simulink model "RT_AI"  (R2024b)
settings: Solver=ode1  StartTime=0.0  StopTime=3  FixedStep=Ts  RelTol=1e-3
PreLoadFcn:
  | Net_improve_init;L=Lac_MV;Tctrl=Ts;
PostLoadFcn:
  | Net_improve_init;L=Lac_MV;Tctrl=Ts;
InitFcn:
  | Net_improve_init;L=Lac_MV;Tctrl=Ts;
undefined symbols (not defined in the file): C1, dend, DiscIntNeverNeededParam, f_cari, fs, Lac_MV, numd, Pref, Rac_MV, Ts, Vac_peak_MV, Vdc
libraries: rtlab x6, spsControlledVoltageSourceLib x6, powerlib_extras x5, artemis x3, spsControlledCurrentSourceLib x3, spsGroundLib x3, simulink x3, spsCurrentMeasurementLib x2, spsThreePhaseVIMeasurementLib x1, spsIdealSwitchLib x1, spsPower3phInstantaneousLib x1, spsSeriesRLCBranchLib x1
Description:
  | The Model initialization function Callback automatically
  | 
  | sets the sample time  to 2e-6 sec.  and loads the initial
  | 
  | states vector xInitial. The initial state vector is saved in the
  | 
  | power_acdrive_init.mat file.
  | 
  | 
  | 
  | Check  the Initial state checkbox in the Simulation
  | 
  | parameters/Workspace I/O to start in steady state with a
  | 
  | speed of 120 rad/s and a torque of 0 N.m/s,
  | 
  | 
  | Copyright 2008-2015 The MathWorks, Inc.
settings Model: Creator=WeiLi  LastModifiedBy=KeXing
settings SolverCC: AlgebraicLoopSolver=TrustRegion
settings DataIOCC: SaveFinalState=on  SaveFormat=Array  SignalLoggingSaveFormat=ModelDataLogs  SaveOutput=off  SaveTime=off  ReturnWorkspaceOutputs=off  SignalLoggingName=sigsOut
settings OptimizationCC: BlockReduction=off  ExpressionDepthLimit=2147483647  InitFltsAndDblsToZero=on  LifeSpan=inf
settings DebuggingCC: SaveWithParameterizedLinksMsg=none  UnderspecifiedInitializationDetection=Classic  MergeDetectMultiDrivingBlocksExec=none  CheckExecutionContextPreStartOutputMsg=on  SignalResolutionControl=TryResolveAllWithWarning  MultiTaskDSMMsg=warning  MultiTaskCondExecSysMsg=none  FcnCallInpInsideContextMsg=warning  UnconnectedInputMsg=warning  UnconnectedLineMsg=warning  StateNameClashWarn=warning  SFUnexpectedBacktrackingDiag=warning  SFNoUnconditionalDefaultTransitionDiag=warning  SFExecutionAtInitializationDiag=none  ArithmeticOperatorsInVariantConditions=warning
settings HardwareCC: ProdBitPerPointer=32  ProdBitPerSizeT=32  ProdBitPerPtrDiffT=32  ProdLargestAtomicFloat=None  ProdIntDivRoundTo=Undefined  ProdEndianess=Unspecified  ProdWordSize=32  ProdHWDeviceType=32-bit Generic  TargetUnknown=on
settings ModelReferenceCC: EnableRefExpFcnMdlSchedulingChecks=on  PropagateSignalLabelsOutOfModel=off
settings SFSimCC: SimUseLocalCustomCode=off  CustomCodeUndefinedFunction=UseInterfaceOnly
settings RTWCC: RTWUseLocalCustomCode=off  GPUComputeCapability=3.5
settings CodeAppCC: StateflowObjectComments=on
settings GRTTargetCC: TargetFcnLib=ansi_tfl_tmw.mat  TargetLangStandard=C89/C90 (ANSI)  CombineOutputUpdateFcns=off  GRTInterface=on
settings ConfigComp: CovMetricSettings=dw  CovSaveCumulativeToWorkspaceVar=on  CovSaveSingleToWorkspaceVar=on  CovExternalEMLEnable=off
settings SimscapeCC: SimscapeNormalizeSystem=off

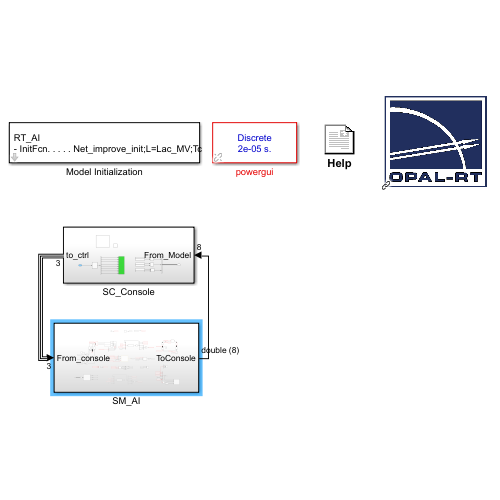
[thumbnail: Simulink's stored preview of the top-level diagram]
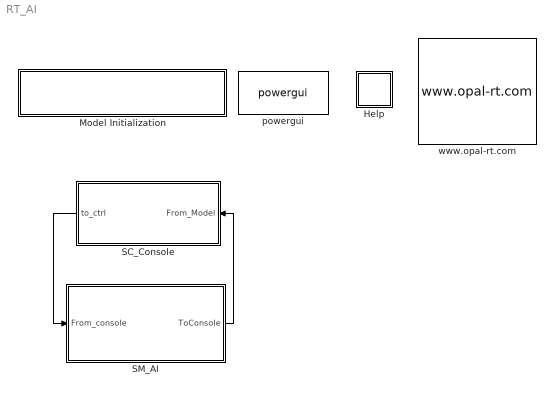
== system RT_AI ==
  Help : Subsystem  mask(OpDoc){docfile=../Help/help.html}
      mask init:
      | %patch([1,1,0,0,.8,1],[.8,0,0,1,1,.8],[.8 .8 .8]);
      | %patch([.15 .78 .78 .15 .15],[.8 .8 .83 .83 .8],[.9 .9 .9]);
      | %patch([.15 .78 .78 .15 .15],[.7 .7 .73 .73 .8],[.9 .9 .9]);
      | %patch([.15 .78 .78 .15 .15],[.6 .6 .63 .63 .6],[.9 .9 .9]);
      | %patch([.15 .78 .78 .15 .15],[.5 .5 .53 .53 .5],[.9 .9 .9]);
      | %patch([.15 .78 .78 .15 .15],[.4 .4 .43 .43 .4],[.9 .9 .9]);
      settings: OpenFcn=OpHelp_cb(gcb);
      mask Display: image(imread('opdoc.bmp'))
  Model Initialization : Subsystem  mask(Model Functions){InitFcnX=Net_improve_init;L=Lac_MV;Tctrl=Ts;, prel=on, posl=on, inif=on, strf=off}
      mask prompts: InitFcnX "Initialisation"; prel "Preload Function"; posl "PostLoad Function"; inif "InitFcn"; strf "StartFcn"
      mask init:
      | currentBlock = gcb;
      | root = bdroot(currentBlock);
      | 
      | if ~strcmp(get_param(root,'BlockDiagramType'),'library')
      |     if prel==1
      |         set_param(root, 'PreLoadFcn', InitFcnX);
      |     else
      |         set_param(root, 'PreLoadFcn', '');
      |     end
      |     if inif==1
      |         set_param(root, 'InitFcn', InitFcnX);
      |     else
      |         set_param(root, 'InitFcn', '');
      |     end
      |     if strf==1
      |         set_param(root, 'StartFcn', InitFcnX);
      |     else
      |         set_param(root, 'StartFcn', '');
      |     end
      |     if posl==1
      |         set_param(root, 'PostLoadFcn', InitFcnX);
      |     else
      |         set_param(root, 'PostLoadFcn', '');
      |     end
      | end
      | 
      | pos = get_param(currentBlock, 'Position');
      | width = pos(3) - pos(1); height = pos(4) - pos(2);
      | txt = [ upper(root) '\n' '- InitFcn. . . . . '  get_param(root, 'InitFcn') ];
      settings: CopyFcn=set_param(gcb,'LinkStatus','none')
      mask Display: text(5, height*0.5, txt, 'horizontalAlignment', 'left', 'verticalAlignment', 'middle') ;
  SC_Console : Subsystem
  SM_AI : Subsystem
  powergui : sps_lib/powergui  Priority=2  SimulationMode=Discrete  SampleTime=Ts  frequency=60  Iterations=50  frequencyindice=0  Pbase=100e6  ErrMax=1e-4  UnitsV=kV  UnitsW=MW  buscounter=0  FunctionMessages=off  echomessages=off  EnableUseOfTLC=off  CurrentSourceSwitches=off  DisableSnubberDevices=off  DisableRonSwitches=off  DisableVfSwitches=off  DisplayEquations=off  AutomaticDiscreteSolvers=off  SolverType=Backward Euler  Interpol=off  ExternalGateDelay=off  methode=off  Ts=0  x0status=blocks  SPID=off  SwTol=0  HookPort=off  NonlinearTolerance=1e-4  nMaxIteration=100  ContinueOnMaxIteration=off  RestoreLinks=warning  ResistiveCurrentMeasurement=off  Frange=[0:2:500]  Ylog=off  Xlog=on  ShowGrid=off  save=off  variable=ZData  structure=VI  ZoomFFT=off  StartTime=9  cycles=10  DisplayStyle=2  fundamental=300/pi  FreqAxis=off  MaxFrequency=1000  frequencyindicesteady=1  RmsSteady=1  display=off
  www.opal-rt.com : artemis/Internal/www.opal-rt.com  SystemSampleTime=-1  VariantActivationTime=update diagram  AllowFlexibleInterface=on  Latency=0  AutoFrameSizeCalculation=off
      settings: SourceProductName=Artemis
  wires:
  SC_Console/1(to_ctrl) -> SM_AI/1(From_console)
  SM_AI/1(ToConsole) -> SC_Console/1(From_Model)

== system RT_AI/Help ==

== system RT_AI/Model Initialization ==

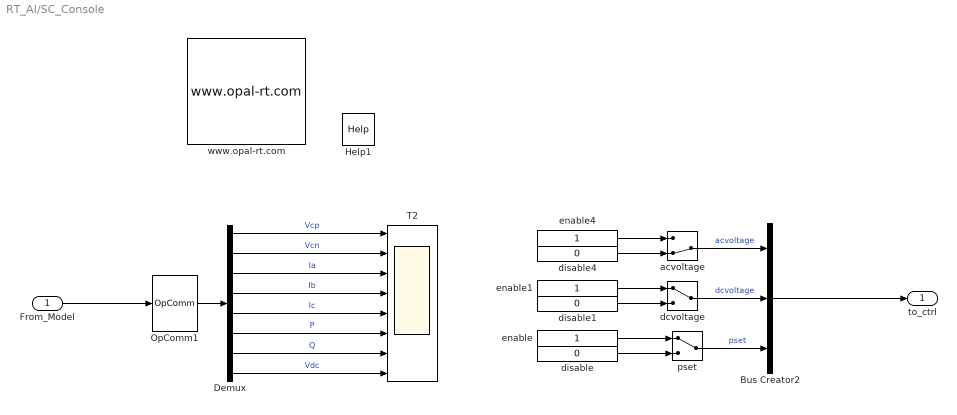
== system RT_AI/SC_Console ==
  From_Model : Inport
  Bus Creator2 : BusCreator  Inputs=3
  Demux : Demux  Outputs=8
  Help1 : artemis/Internal/Help  docfile=../help/help.html
      settings: SourceProductName=Artemis
  OpComm1 : rtlab/OpComm  nbport=1  groupe_acq=1  subsys_rate=Ts  st=0  Synchronization=off  Interpolation=on  Threshold=1.0  Missed_Data=off  Sim_Time=off  Samples=off  dynSigOut=off  from_console=0  warning_done=off  writeOpCommFile=off  Offset=off
      settings: SourceProductName=RT-LAB
  T2 : Scope  NumInputPorts=8
  acvoltage : ManualSwitch  CurrentSetting=0
  dcvoltage : ManualSwitch
  disable : Constant  Value=0
  disable1 : Constant  Value=0
  disable4 : Constant  Value=0
  enable : Constant
  enable1 : Constant
  enable4 : Constant
  pset : ManualSwitch
  www.opal-rt.com : artemis/Internal/www.opal-rt.com  SystemSampleTime=-1  VariantActivationTime=update diagram  AllowFlexibleInterface=on  Latency=0  AutoFrameSizeCalculation=off
      settings: SourceProductName=Artemis
  to_ctrl : Outport
  wires:
  enable/1 -> pset/1
  Bus Creator2/1 -> to_ctrl/1
  dcvoltage/1 -> Bus Creator2/2  "dcvoltage"
  disable1/1 -> dcvoltage/2
  disable/1 -> pset/2
  enable1/1 -> dcvoltage/1
  disable4/1 -> acvoltage/2
  enable4/1 -> acvoltage/1
  acvoltage/1 -> Bus Creator2/1  "acvoltage"
  pset/1 -> Bus Creator2/3  "pset"
  Demux/1 -> T2/1  "Vcp"
  Demux/6 -> T2/6  "P"
  From_Model/1 -> OpComm1/1
  Demux/2 -> T2/2  "Vcn"
  OpComm1/1 -> Demux/1
  Demux/3 -> T2/3  "Ia"
  Demux/8 -> T2/8  "Vdc"
  Demux/4 -> T2/4  "Ib"
  Demux/5 -> T2/5  "Ic"
  Demux/7 -> T2/7  "Q"

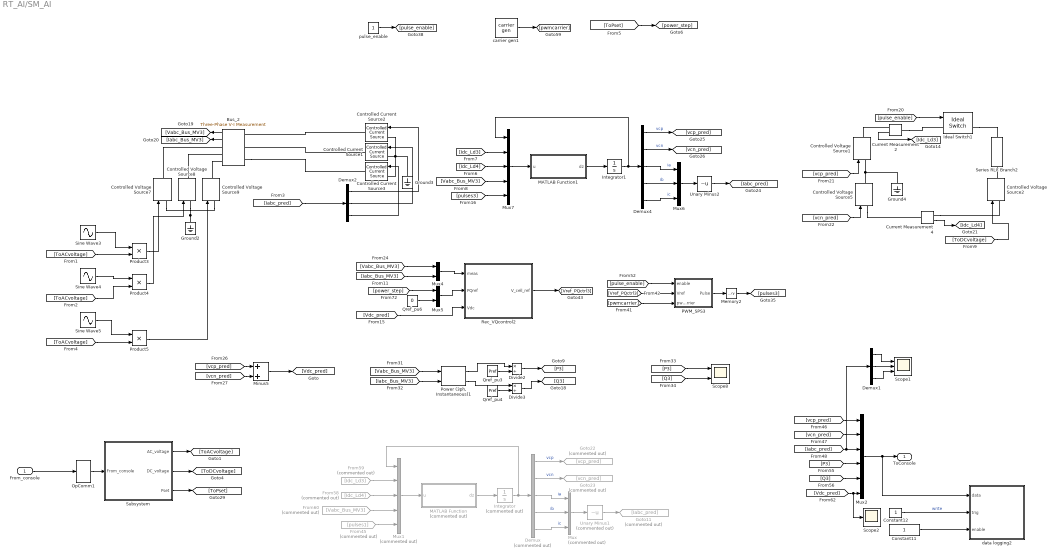
== system RT_AI/SM_AI ==
  From_console : Inport
  Bus_2 : spsThreePhaseVIMeasurementLib/Three-Phase V-I Measurement  VoltageMeasurement=phase-to-ground  SetLabelV=off  LabelV=Vabc  Vpu=off  VpuLL=off  CurrentMeasurement=yes  SetLabelI=off  LabelI=Iabc  Ipu=off  Pbase=P_AC  Vbase=V_AC_prim  OutputType=Complex  PhasorSimulation=off  PSBequivalent=0
  Constant11 : Constant
  Constant12 : Constant
  Controlled Current Source1 : spsControlledCurrentSourceLib/Controlled Current Source  Initialize=on  Source_Type=AC  Amplitude=0  Phase=0  Frequency=0  Measurements=None
  Controlled Current Source2 : spsControlledCurrentSourceLib/Controlled Current Source  Initialize=on  Source_Type=AC  Amplitude=0  Phase=0  Frequency=0  Measurements=None
  Controlled Current Source3 : spsControlledCurrentSourceLib/Controlled Current Source  Initialize=on  Source_Type=AC  Amplitude=0  Phase=0  Frequency=0  Measurements=None
  Controlled Voltage Source1 : spsControlledVoltageSourceLib/Controlled Voltage Source  Initialize=on  Source_Type=DC  Amplitude=3000  Phase=0  Frequency=0  Measurements=None
  Controlled Voltage Source2 : spsControlledVoltageSourceLib/Controlled Voltage Source  Initialize=on  Source_Type=DC  Amplitude=3000  Phase=0  Frequency=0  Measurements=None
  Controlled Voltage Source5 : spsControlledVoltageSourceLib/Controlled Voltage Source  Initialize=on  Source_Type=DC  Amplitude=3000  Phase=0  Frequency=0  Measurements=None
  Controlled Voltage Source7 : spsControlledVoltageSourceLib/Controlled Voltage Source  Initialize=off  Source_Type=AC  Amplitude=0  Phase=0  Frequency=fs  Measurements=None
  Controlled Voltage Source8 : spsControlledVoltageSourceLib/Controlled Voltage Source  Initialize=off  Source_Type=AC  Amplitude=0  Phase=0  Frequency=fs  Measurements=None
  Controlled Voltage Source9 : spsControlledVoltageSourceLib/Controlled Voltage Source  Initialize=off  Source_Type=AC  Amplitude=0  Phase=0  Frequency=fs  Measurements=None
  Current Measurement2 : spsCurrentMeasurementLib/Current Measurement  PhasorSimulation=off  OutputType=Complex  PSBequivalent=0
  Current Measurement4 : spsCurrentMeasurementLib/Current Measurement  PhasorSimulation=off  OutputType=Complex  PSBequivalent=0
  Demux : Demux  Commented=on  Outputs=5
  Demux1 : Demux  Outputs=3
  Demux2 : Demux  Outputs=3
  Demux4 : Demux  Outputs=5
  Divide2 : Product  Inputs=*/
  Divide3 : Product  Inputs=*/
  From45 : From  Commented=on  GotoTag=pulses1
  From58 : From  Commented=on  GotoTag=Idc_Ld4
  From59 : From  Commented=on  GotoTag=Idc_Ld3
  From60 : From  Commented=on  GotoTag=Vabc_Bus_MV3
  Goto11 : Goto  Commented=on  GotoTag=Iabc_pred
  Goto22 : Goto  Commented=on  GotoTag=vcp_pred
  Goto23 : Goto  Commented=on  GotoTag=vcn_pred
  Ground2 : spsGroundLib/Ground  LConnTagsString=a
  Ground3 : spsGroundLib/Ground  LConnTagsString=a
  Ground4 : spsGroundLib/Ground  LConnTagsString=a
  Ideal Switch1 : spsIdealSwitchLib/Ideal Switch  Ron=0.001  Lon=0  IC=0  Rs=1e9  Cs=inf  Measurements=on
  Integrator : Integrator  Commented=on
  Integrator1 : Integrator
  MATLAB Function : MATLAB Function  Commented=on  TreatAsAtomicUnit=on
  MATLAB Function1 : MATLAB Function  TreatAsAtomicUnit=on
  Memory2 : Memory
  Minus5 : Sum
  Mux : Mux  Commented=on  Inputs=3
  Mux1 : Mux  Commented=on  Inputs=5
  Mux2 : Mux  Inputs=6
  Mux4 : Mux  Inputs=2
  Mux5 : Mux  Inputs=2
  Mux6 : Mux  Inputs=3
  Mux7 : Mux  Inputs=5
  OpComm1 : rtlab/OpComm  nbport=1  groupe_acq=1  subsys_rate=Ts  st=0  Synchronization=on  Interpolation=on  Threshold=1.0  Missed_Data=off  Sim_Time=off  Samples=off  dynSigOut=off  from_console=1  warning_done=off  writeOpCommFile=off  Offset=off
      settings: SourceProductName=RT-LAB
  PWM_SPS3 : Subsystem
  "Power (3ph, Instantaneous)1" : spsPower3phInstantaneousLib/Power (3ph, Instantaneous)
  Product3 : Product
  Product4 : Product
  Product5 : Product
  Qref_pu3 : Constant  Value=Pref
  Qref_pu4 : Constant  Value=Pref
  Qref_pu6 : Constant  Value=0
  Rec_VQcontrol2 : Subsystem  mask(converter controller){cm=off, base=[Pref, Vac_peak_MV*sqrt(3/2), Vdc/2, fs], LRx=[Lac_MV, Rac_MV], LRx_inpu=off, Kd=[0.3  2]*10/6  %was [1 0.1]   ; [0.1  1]*1, Kp=[0.3 1]*1     %was [1 0.1]   ; [0.1  1]*1, Kvdc=[2 10]*1;   %was [0.5 1]*20 for Cdc=320uF, Vabc_lim=[-1 1], limitVdq=1.1, nadv=6, xtrIctrl1=[0.4 10 10 -10], Ts=Tctrl}
      mask prompts: cm "control mode (check VQ/uncheck PQ), only one terminal in VQ mode"; base "base value for power(VA), ac voltage(V), dc voltage to ground(V), and frequenvy(Hz) [Sb, Vb, Vdcb,freq]"; LRx "commutation inductance and resistance [Lx, Rx]"; LRx_inpu "[Lx, Rx] in pu if checked/ SI unchecked"; Kd "Kp Ki for d-axis PI control [kp ki]"; Kp "Kp Ki for q-axis PI control [kp ki]"; Kvdc "Kp Ki for Vdc PI control [kp ki]"; Vabc_lim "output Vabc limit [min max]"; limitVdq "limit for Vd,Vq (pu, default = 1.1)"; nadv "nb of time step to compesate for delay (default=1)"; xtrIctrl1 "[kp, kp, limitmax, limitmin] for current control (default=[0.4, 10, 10, -10])"
      mask help:
      | input 1, 6 dimentions, Vabc, Iabc, (SI)
      | input 2, 2 dimentions, Pref, Qref (PU)
      | input 3, 6 dimentions, Vcap at up arm a, lower arm a, up arm b, lower arm b, up arm c and lower arm c.
      | input 4, 1 dimention, pulse on
      | input 5, 1 dimention
      |
      | power or current directions: to go into grid is positive
      mask init:
      | if cm==0;
      |     x=['PQ\nmode'];
      | else
      |     x=['VQ\nmode'];
      | end
      | 
      | Sb=base(1);            %VA 3phase power base;
      | Vb=base(2);       %V, line-line rms voltage base
      | Ib=Sb/(sqrt(3)*Vb); %A, rms current base
      | Zb=Vb^2/Sb ;        %ohm, impedence base
      | Vdc=base(3);      %V Vdc+ to ground or ground to Vdc- 
      | frq=base(4);
      | 
      | if LRx_inpu
      |     Rxpu=LRx(2);
      |     Lxpu=LRx(1);
      | else
      |     Rxpu=LRx(2)/Zb;
      |     Lxpu=LRx(1)*2*pi*frq/Zb;
      | end;
      | 
      | ks=Vdc*sqrt(3/2)/Vb;     % ma=1/ks for 1pu dc ->1pu ac;
      | 
      | Kp=Kd;
      mask DialogControl ParameterTabVar0 Prompt: parameters
      mask DialogControl ParameterTabVar01 Prompt: advanced
      mask Display: disp (x);
  Scope1 : Scope  NumInputPorts=3
  Scope2 : Scope
  Scope8 : Scope  NumInputPorts=2
  Series RLC Branch2 : spsSeriesRLCBranchLib/Series RLC Branch  LConnTagsString=__new0  RConnTagsString=__new0  BranchType=R  Resistance=3e3^2/(Pref)/10*2  Inductance=1e-3  SetiL0=off  InitialCurrent=0  Capacitance=C1  Setx0=off  InitialVoltage=0  Measurements=None
  Sine Wave3 : Sin  Amplitude=3e3/2*sqrt(2/3)  Frequency=2*pi*fs  SampleTime=0
  Sine Wave4 : Sin  Amplitude=3e3/2*sqrt(2/3)  Frequency=2*pi*fs  Phase=-2*pi/3  SampleTime=0
  Sine Wave5 : Sin  Amplitude=3e3/2*sqrt(2/3)  Frequency=2*pi*fs  Phase=+2*pi/3  SampleTime=0
  Subsystem : Subsystem
  Unary Minus1 : UnaryMinus  Commented=on
  Unary Minus2 : UnaryMinus
  carrier gen1 : libMMCcpuv2/carrier gen  fc=f_cari*2  range=[ 1 -1]  Ms=3  Ns=1
  data logging2 : Subsystem
  pulse_enable : Constant
  ToConsole : Outport
  wires:
  Subsystem/3(Pset) -> [ToPset]
  Demux/1 -> Goto22/1  "vcp"
  Qref_pu4/1 -> Divide3/2
  [pulse_enable] -> PWM_SPS3/1(enable)
  Bus_2/1 -> [Vabc_Bus_MV3]
  Bus_2/2 -> [Iabc_Bus_MV3]
  Subsystem/1(AC_voltage) -> [ToACvoltage]
  Unary Minus1/1 -> Goto11/1
  pulse_enable/1 -> [pulse_enable]
  Demux4/5 -> Mux6/3  "ic"
  Subsystem/2(DC_voltage) -> [ToDCvoltage]
  From60/1 -> Mux1/4
  [Vdc_pred] -> Scope2/1, Mux2/6
  From_console/1 -> OpComm1/1
  Demux2/3 -> Controlled Current Source3/1
  [vcp_pred] -> Minus5/1
  [ToACvoltage] -> Product5/2
  [Q3] -> Scope8/2
  [pulse_enable] -> Ideal Switch1/1
  PWM_SPS3/1(Pulse) -> Memory2/1
  [vcp_pred] -> Controlled Voltage Source1/1
  Demux/2 -> Goto23/1  "vcn"
  Product5/1 -> Controlled Voltage Source9/1
  [vcp_pred] -> Mux2/1
  [Iabc_pred] -> Demux2/1
  Mux1/1 -> MATLAB Function/1(u)
  Demux/4 -> Mux/2  "ib"
  [ToACvoltage] -> Product3/2
  [Vabc_Bus_MV3] -> Mux7/4
  Mux7/1 -> MATLAB Function1/1(u)
  [ToDCvoltage] -> Controlled Voltage Source2/1
  [vcn_pred] -> Mux2/2
  Sine Wave3/1 -> Product3/1
  Current Measurement4/1 -> [Idc_Ld4]
  [P3] -> Scope8/1
  "Power (3ph, Instantaneous)1"/2 -> Divide3/1
  [power_step] -> Mux5/1
  Demux4/4 -> Mux6/2  "ib"
  Product4/1 -> Controlled Voltage Source8/1
  [Vabc_Bus_MV3] -> "Power (3ph, Instantaneous)1"/1
  Integrator1/1 -> Mux7/1, Demux4/1
  [Idc_Ld3] -> Mux7/2
  Divide3/1 -> [Q3]
  Product3/1 -> Controlled Voltage Source7/1
  [ToPset] -> [power_step]
  [pwmcarrier] -> PWM_SPS3/3(pwmcarrier)
  Demux2/2 -> Controlled Current Source1/1
  [P3] -> Mux2/4
  [Vref_PQctrl3] -> PWM_SPS3/2(Vref)
  Unary Minus2/1 -> [Iabc_pred]
  Demux/5 -> Mux/3  "ic"
  Demux4/3 -> Mux6/1  "ia"
  Sine Wave4/1 -> Product4/1
  Sine Wave5/1 -> Product5/1
  Memory2/1 -> [pulses3]
  [Iabc_pred] -> Demux1/1, Mux2/3
  Integrator/1 -> Mux1/1, Demux/1
  Qref_pu3/1 -> Divide2/2
  [Vdc_pred] -> Rec_VQcontrol2/3(Vdc)
  [Vabc_Bus_MV3] -> Mux4/1
  Qref_pu6/1 -> Mux5/2
  MATLAB Function1/1(dz) -> Integrator1/1
  Rec_VQcontrol2/1(V_cell_ref) -> [Vref_PQctrl3]
  [vcn_pred] -> Minus5/2
  Current Measurement2/1 -> [Idc_Ld3]
  [Q3] -> Mux2/5
  [Idc_Ld4] -> Mux7/3
  Mux/1 -> Unary Minus1/1
  [vcn_pred] -> Controlled Voltage Source5/1
  Demux4/2 -> [vcn_pred]  "vcn"
  From58/1 -> Mux1/3
  MATLAB Function/1(dz) -> Integrator/1
  "Power (3ph, Instantaneous)1"/1 -> Divide2/1
  From59/1 -> Mux1/2
  Demux2/1 -> Controlled Current Source2/1
  Demux/3 -> Mux/1  "ia"
  Mux6/1 -> Unary Minus2/1
  [ToACvoltage] -> Product4/2
  [Iabc_Bus_MV3] -> Mux4/2
  [Iabc_Bus_MV3] -> "Power (3ph, Instantaneous)1"/2
  From45/1 -> Mux1/5
  Mux5/1 -> Rec_VQcontrol2/2(PQref)
  Minus5/1 -> [Vdc_pred]
  [pulses3] -> Mux7/5
  Divide2/1 -> [P3]
  carrier gen1/1 -> [pwmcarrier]
  Demux4/1 -> [vcp_pred]  "vcp"
  Mux4/1 -> Rec_VQcontrol2/1(meas)
  OpComm1/1 -> Subsystem/1(From_console)
  Constant12/1 -> data logging2/2(trig)  "write"
  Constant11/1 -> data logging2/3(enable)
  Mux2/1 -> data logging2/1(data), ToConsole/1
  Demux1/1 -> Scope1/1
  Demux1/2 -> Scope1/2
  Demux1/3 -> Scope1/3
  connections:
  Controlled Voltage Source5/RConn1 -- Ground4/LConn1 -- Controlled Voltage Source1/LConn1
  Ground2/LConn1 -- Controlled Voltage Source9/LConn1 -- Controlled Voltage Source7/LConn1 -- Controlled Voltage Source8/LConn1
  Current Measurement2/LConn1 -- Ideal Switch1/LConn1
  Controlled Current Source2/RConn1 -- Bus_2/LConn1
  Controlled Voltage Source5/LConn1 -- Current Measurement4/LConn1
  Bus_2/RConn2 -- Controlled Voltage Source8/RConn1
  Ideal Switch1/RConn1 -- Series RLC Branch2/RConn1
  Current Measurement4/RConn1 -- Controlled Voltage Source2/LConn1
  Bus_2/RConn1 -- Controlled Voltage Source7/RConn1
  Bus_2/RConn3 -- Controlled Voltage Source9/RConn1
  Controlled Current Source2/LConn1 -- Ground3/LConn1 -- Controlled Current Source3/LConn1 -- Controlled Current Source1/LConn1
  Bus_2/LConn3 -- Controlled Current Source3/RConn1
  Current Measurement2/RConn1 -- Controlled Voltage Source1/RConn1
  Controlled Current Source1/RConn1 -- Bus_2/LConn2
  Controlled Voltage Source2/RConn1 -- Series RLC Branch2/LConn1

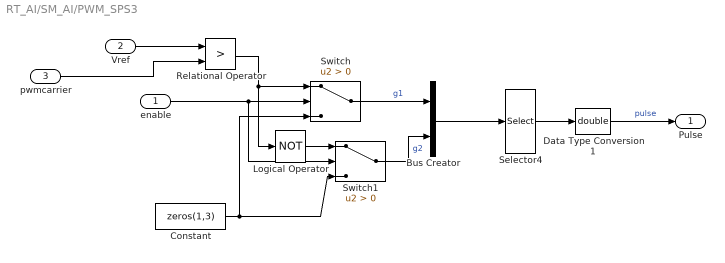
== system RT_AI/SM_AI/PWM_SPS3 ==
  enable : Inport
  Vref : Inport  Port=2
  pwmcarrier : Inport  Port=3
  Bus Creator : BusCreator  Inputs=2
  Constant : Constant  Value=zeros(1,3)
  Data Type Conversion1 : DataTypeConversion  OutDataTypeStr=double  SaturateOnIntegerOverflow=off  RndMeth=Floor
  Logical Operator : Logic  Operator=NOT  AllPortsSameDT=off  OutDataTypeStr=boolean
  Relational Operator : RelationalOperator  Operator=>  OutDataTypeStr=boolean  InputSameDT=off
  Selector4 : Selector  InputPortWidth=6  IndexOptions=Index vector (dialog)  Indices=[1 4 2 5 3 6]  OutputSizes=1
  Switch : Switch  Criteria=u2 > Threshold  SaturateOnIntegerOverflow=off  InputSameDT=off
  Switch1 : Switch  Criteria=u2 > Threshold  SaturateOnIntegerOverflow=off  InputSameDT=off
  Pulse : Outport  VectorParamsAs1DForOutWhenUnconnected=off
  wires:
  Data Type Conversion1/1 -> Pulse/1  "pulse"
  Bus Creator/1 -> Selector4/1
  Selector4/1 -> Data Type Conversion1/1
  Constant/1 -> Switch1/3, Switch/3
  Logical Operator/1 -> Switch1/1
  Switch1/1 -> Bus Creator/2  "g2"
  Switch/1 -> Bus Creator/1  "g1"
  Relational Operator/1 -> Switch/1, Logical Operator/1
  enable/1 -> Switch/2, Switch1/2
  pwmcarrier/1 -> Relational Operator/2
  Vref/1 -> Relational Operator/1

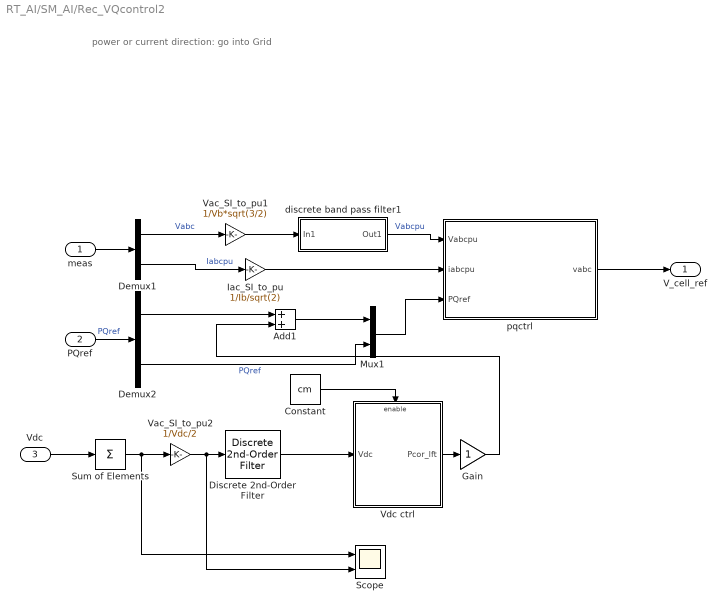
== system RT_AI/SM_AI/Rec_VQcontrol2 ==
  note: power or current direction: go into Grid
  meas : Inport
  PQref : Inport  Port=2
  Vdc : Inport  Port=3
  Add1 : Sum
  Constant : Constant  Value=cm
  Demux1 : Demux  Outputs=[3 3 ]
  Demux2 : Demux  Outputs=2
  Discrete 2nd-Order Filter : powerlib_extras/Discrete  Control Blocks/Discrete  2nd-Order Filter  FilterType=Lowpass  Fo=90  Zeta=0.707  Ts=Ts  Initialize=off  Vac_Init=[0.8 -25 60]  Vdc_Init=-0.4  PlotResponse=off  param1=[1 500 1]
  Gain : Gain
  Iac_SI_to_pu : Gain  Gain=1/Ib/sqrt(2)
  Mux1 : Mux  Inputs=2
  Scope : Scope  NumInputPorts=2
  Sum of Elements : Sum  Inputs=+
  Vac_SI_to_pu1 : Gain  Gain=1/Vb*sqrt(3/2)
  Vac_SI_to_pu2 : Gain  Gain=1/Vdc/2  SampleTime=Ts
  Vdc ctrl : Subsystem
  discrete band pass filter1 : Subsystem  mask(discrete transfer Fcn generator){Fo=frq, adj1=1, inistate=0, Ts=Ts, bodedw=off}
      mask prompts: Fo "F0 (Hz)"; adj1 "adj (1 for no adjustment, larger adj for wider band pass)"; inistate "Initial states"; Ts "Sample time (must be explicite)"; bodedw "draw Bode diagram of filter"
      mask help:
      | This block transfer a continous TF to a discrete TF
      | using Bilinear (Tustin) approximation
      mask init:
      | AD1=tf([1 0],1);
      | 
      | %second order
      | % Fo=50; %cut off freq.
      | % omega0=Fo*2*pi;
      | % adj1=3;   %adjustment 1
      | Zeta= 0.707*adj1; %Damping factor Zeta ( Q = 1 / (2*Zeta) ):
      | Wo=2*pi*Fo;
      | % str=sprintf(' Fo=%iHz\n\n',Fo);
      |  n2=0; n1=0;n0=Wo*Wo;
      |  d2=1;d1=2*Zeta*Wo;d0=Wo*Wo;
      | numc=[n2 n1 n0];
      | denc=[d2 d1 d0];
      | AD3=tf(numc,denc);
      | 
      | AD4=AD1*AD3;
      | [mag1,pha1]=bode(AD4,Wo);
      | mag0=mag1;
      | AD=AD4/mag0;
      | 
      | if bodedw==1
      |     figure;
      |     h=bodeplot(AD1,AD3,AD);
      |     setoptions(h,'FreqUnits','Hz');
      |     grid on;
      |     title(['Bode Diagram, adj=',num2str(adj1)]);
      | end;
      |     
      | % gg=tf(num,den);
      | ggd=c2d(AD,Ts,'tustin');
      | [numd,dend] = tfdata(ggd,'v');
  pqctrl : Subsystem
  V_cell_ref : Outport  VectorParamsAs1DForOutWhenUnconnected=off
  wires:
  Constant/1 -> Vdc ctrl/Enable
  Vac_SI_to_pu1/1 -> discrete band pass filter1/1(In1)
  Vac_SI_to_pu2/1 -> Scope/2, Discrete 2nd-Order Filter/1
  Vdc/1 -> Sum of Elements/1
  Discrete 2nd-Order Filter/1 -> Vdc ctrl/1(Vdc)
  Mux1/1 -> pqctrl/3(PQref)
  Demux2/2 -> Mux1/2  "PQref"
  Add1/1 -> Mux1/1
  Vdc ctrl/1(Pcor_lft) -> Gain/1
  Demux2/1 -> Add1/1
  Iac_SI_to_pu/1 -> pqctrl/2(iabcpu)
  Demux1/1 -> Vac_SI_to_pu1/1  "Vabc"
  Demux1/2 -> Iac_SI_to_pu/1  "Iabcpu"
  meas/1 -> Demux1/1
  discrete band pass filter1/1(Out1) -> pqctrl/1(Vabcpu)  "Vabcpu"
  PQref/1 -> Demux2/1  "PQref"
  pqctrl/1(vabc) -> V_cell_ref/1
  Sum of Elements/1 -> Scope/1, Vac_SI_to_pu2/1
  Gain/1 -> Add1/2

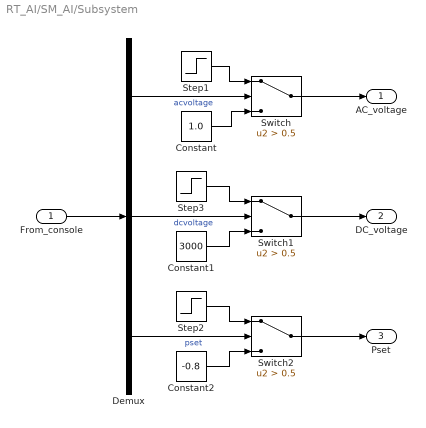
== system RT_AI/SM_AI/Subsystem ==
  From_console : Inport
  Constant : Constant  Value=1.0
  Constant1 : Constant  Value=3000
  Constant2 : Constant  Value=-0.8
  Demux : Demux  Outputs=3
  Step1 : Step  Time=2.5  Before=1.0  After=0.7  SampleTime=0
  Step2 : Step  Time=1.5  Before=-0.8  After=-0.6  SampleTime=0
  Step3 : Step  Time=0.5  Before=3000  After=3200  SampleTime=0
  Switch : Switch  Criteria=u2 > Threshold  Threshold=0.5  SaturateOnIntegerOverflow=off  InputSameDT=off
  Switch1 : Switch  Criteria=u2 > Threshold  Threshold=0.5  SaturateOnIntegerOverflow=off  InputSameDT=off
  Switch2 : Switch  Criteria=u2 > Threshold  Threshold=0.5  SaturateOnIntegerOverflow=off  InputSameDT=off
  AC_voltage : Outport
  DC_voltage : Outport  Port=2
  Pset : Outport  Port=3
  wires:
  Step3/1 -> Switch1/1
  Switch/1 -> AC_voltage/1
  Switch1/1 -> DC_voltage/1
  Step2/1 -> Switch2/1
  Demux/3 -> Switch2/2  "pset"
  Constant1/1 -> Switch1/3
  Step1/1 -> Switch/1
  Switch2/1 -> Pset/1
  Constant/1 -> Switch/3
  Demux/2 -> Switch1/2  "dcvoltage"
  From_console/1 -> Demux/1
  Demux/1 -> Switch/2  "acvoltage"
  Constant2/1 -> Switch2/3

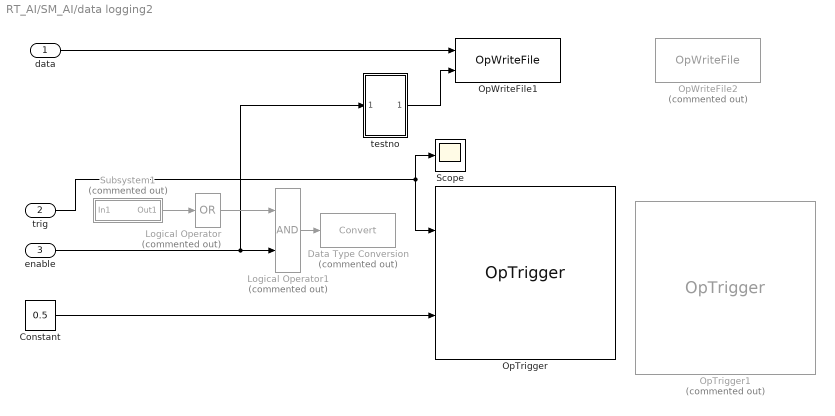
== system RT_AI/SM_AI/data logging2 ==
  data : Inport
  trig : Inport  Port=2
  enable : Inport  Port=3
  Constant : Constant  Value=0.5
  Data Type Conversion : DataTypeConversion  Commented=on  SaturateOnIntegerOverflow=off  RndMeth=Floor
  Logical Operator : Logic  Commented=on  Operator=OR  Inputs=1  AllPortsSameDT=off  OutDataTypeStr=boolean
  Logical Operator1 : Logic  Commented=on  AllPortsSameDT=off  OutDataTypeStr=boolean
  OpTrigger : rtlab/DataLogging/OpTrigger  Trig_Type=TRIGGER SIGNAL >= TRIGGER LEVEL  Trig_Offset=-2000  Acq_Group=27
      settings: SourceProductName=RT-LAB
  OpTrigger1 : rtlab/DataLogging/OpTrigger  Commented=on  Trig_Type=RISING EDGE  Trig_Offset=-1000  Acq_Group=27
      settings: SourceProductName=RT-LAB
  OpWriteFile1 : rtlab/DataLogging/OpWriteFile  Static_File=off  varname=opvar  Filename=1data.mat  rtpath='./'  nrtpath='.\'  Acq_Group=27  file_size=81000000000  write_offline=off  Sim_Mode=off  Nb_Samples=1000  Buffer_size=96000*15*5
      settings: SourceProductName=RT-LAB
  OpWriteFile2 : rtlab/DataLogging/OpWriteFile  Commented=on  Static_File=off  varname=opvar  Filename=2lvl_OPAL.mat  rtpath='./'  nrtpath='.\'  Acq_Group=27  file_size=81000000000  write_offline=off  Sim_Mode=off  Nb_Samples=2048  Buffer_size=163840
      settings: SourceProductName=RT-LAB
  Scope : Scope
  Subsystem1 : Subsystem  Commented=on
  testno : Subsystem
  wires:
  testno/1(Out1) -> OpWriteFile1/2
  Constant/1 -> OpTrigger/2
  enable/1 -> testno/1(In1), Logical Operator1/2
  Logical Operator1/1 -> Data Type Conversion/1
  Subsystem1/1(Out1) -> Logical Operator/1
  Logical Operator/1 -> Logical Operator1/1
  data/1 -> OpWriteFile1/1
  trig/1 -> Scope/1, OpTrigger/1

== system RT_AI/SM_AI/Rec_VQcontrol2/Vdc ctrl ==
  Vdc : Inport
  Enable : EnablePort  StatesWhenEnabling=reset
  Vdc_ctrler1 : Subsystem
  Pcor_lft : Outport  OutputWhenDisabled=reset  InitialOutput=0  VectorParamsAs1DForOutWhenUnconnected=off
  wires:
  Vdc_ctrler1/1(delP) -> Pcor_lft/1  "Pclft"
  Vdc/1 -> Vdc_ctrler1/1(Vcap)

== system RT_AI/SM_AI/Rec_VQcontrol2/discrete band pass filter1 ==
  In1 : Inport
  Discrete Transfer Fcn : DiscreteTransferFcn  Numerator=numd  Denominator=dend  InitialStates=inistate  SampleTime=Ts
  Out1 : Outport  VectorParamsAs1DForOutWhenUnconnected=off
  wires:
  Discrete Transfer Fcn/1 -> Out1/1
  In1/1 -> Discrete Transfer Fcn/1

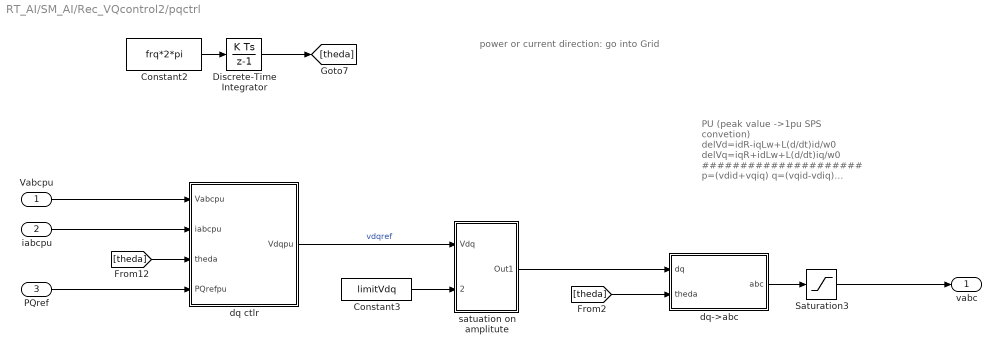
== system RT_AI/SM_AI/Rec_VQcontrol2/pqctrl ==
  note: PU
      | (peak value ->1pu
      | SPS convetion)
      |
      | delVd=idR-iqLw+L(d/dt)id/w0
      | delVq=iqR+idLw+L(d/dt)iq/w0
      | #####################
      | p=(vdid+vqiq)
      | q=(vqid-vdiq)
      | =>
      | Id=(Vd*P+Vq*Q)/C
      | Iq=(Vq*P-Vd*Q)/C
      | C=Vd^2+Vq^2
  note: power or current direction: go into Grid
  Vabcpu : Inport
  iabcpu : Inport  Port=2
  PQref : Inport  Port=3
  Constant2 : Constant  Value=frq*2*pi
  Constant3 : Constant  Value=limitVdq
  Discrete-Time Integrator : DiscreteIntegrator  SampleTime=Ts  ICPrevOutput=DiscIntNeverNeededParam  ICPrevScaledInput=DiscIntNeverNeededParam
  Saturation3 : Saturate  UpperLimit=Vabc_lim(2)  LowerLimit=Vabc_lim(1)
  dq ctlr : Subsystem
  dq->abc : Subsystem
  "satuation on amplitute " : Subsystem
  vabc : Outport  VectorParamsAs1DForOutWhenUnconnected=off
  wires:
  Saturation3/1 -> vabc/1
  [theda] -> dq->abc/2(theda)
  dq->abc/1(abc) -> Saturation3/1
  Constant3/1 -> "satuation on amplitute "/2(limitVdq)
  "satuation on amplitute "/1(Out1) -> dq->abc/1(dq)
  Constant2/1 -> Discrete-Time Integrator/1
  Discrete-Time Integrator/1 -> [theda]
  [theda] -> dq ctlr/3(theda)
  dq ctlr/1(Vdqpu) -> "satuation on amplitute "/1(Vdq)  "vdqref"
  Vabcpu/1 -> dq ctlr/1(Vabcpu)
  iabcpu/1 -> dq ctlr/2(iabcpu)
  PQref/1 -> dq ctlr/4(PQrefpu)

== system RT_AI/SM_AI/data logging2/Subsystem1 ==
  In1 : Inport
  Memory1 : Memory
  Relational Operator : RelationalOperator  Operator=~=  OutDataTypeStr=boolean  InputSameDT=off
  Out1 : Outport  VectorParamsAs1DForOutWhenUnconnected=off
  wires:
  In1/1 -> Memory1/1, Relational Operator/1
  Memory1/1 -> Relational Operator/2
  Relational Operator/1 -> Out1/1

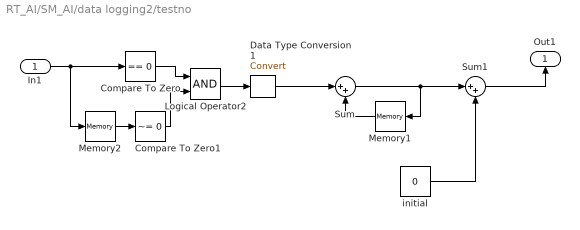
== system RT_AI/SM_AI/data logging2/testno ==
  In1 : Inport
  Compare To Zero : simulink/Logic and Bit Operations/Compare To Zero  relop===  OutDataTypeStr=uint8
  Compare To Zero1 : simulink/Logic and Bit Operations/Compare To Zero  relop=~=  OutDataTypeStr=uint8
  Data Type Conversion1 : DataTypeConversion  SaturateOnIntegerOverflow=off  RndMeth=Floor
  Logical Operator2 : Logic  AllPortsSameDT=off  OutDataTypeStr=boolean
  Memory1 : Memory
  Memory2 : Memory
  Sum : Sum  Inputs=|++
  Sum1 : Sum  Inputs=|++
  initial : Constant  Value=0
  Out1 : Outport  VectorParamsAs1DForOutWhenUnconnected=off
  wires:
  Data Type Conversion1/1 -> Sum/1
  Sum1/1 -> Out1/1
  initial/1 -> Sum1/2
  In1/1 -> Memory2/1, Compare To Zero/1
  Compare To Zero1/1 -> Logical Operator2/2
  Logical Operator2/1 -> Data Type Conversion1/1
  Memory2/1 -> Compare To Zero1/1
  Compare To Zero/1 -> Logical Operator2/1
  Memory1/1 -> Sum/2
  Sum/1 -> Sum1/1, Memory1/1

== system RT_AI/SM_AI/Rec_VQcontrol2/Vdc ctrl/Vdc_ctrler1 ==
  Vcap : Inport
  Add2 : Sum  Inputs=+-
  PI_d2 : Subsystem  AncestorBlock=|  DialogController=POWERSYS.PowerSysDialog  mask(Discrete PI Controller){Kp=Kvdc(1), Ki=Kvdc(2), Par_Limits=[1 -1]*1, Init=0, Ts=Ts}
      | powerlib_extras/Discrete 
      | Control Blocks/Discrete
      | PI Controller
      mask prompts: Kp "Proportional gain (Kp):"; Ki "Integral gain (Ki):"; Par_Limits "Output limits: [ Upper   Lower ]"; Init "Output initial value:"; Ts "Sample time:"
      mask help: This block implements a discrete PI controller.
      mask init:
      | UpperLimit=Par_Limits(1);
      | LowerLimit=Par_Limits(2);
      | power_initmask();
      mask Help: This block is part of a subset of blocks in the Extras library that does not have documentation associated with it, other than the block mask description.
      mask Display: disp('PI');
  Saturation : Saturate  UpperLimit=0.1  LowerLimit=-0.1
      settings: AttributesFormatString=%<LowerLimit>~%<UpperLimit>
  Vdcpuref : Constant
  Vdctrl : Scope  NumInputPorts=2
  delP : Outport  OutputWhenDisabled=reset  InitialOutput=[0]  VectorParamsAs1DForOutWhenUnconnected=off
  wires:
  PI_d2/1(Out) -> delP/1, Vdctrl/2  "PIVdc"
  Saturation/1 -> PI_d2/1(Error)
  Vdcpuref/1 -> Add2/2
  Vcap/1 -> Add2/1, Vdctrl/1
  Add2/1 -> Saturation/1  "delVdc"

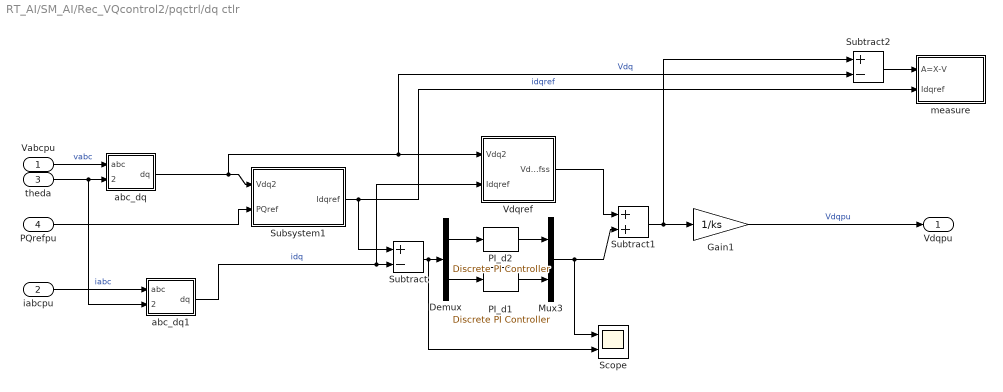
== system RT_AI/SM_AI/Rec_VQcontrol2/pqctrl/dq ctlr ==
  Vabcpu : Inport
  iabcpu : Inport  Port=2
  theda : Inport  Port=3
  PQrefpu : Inport  Port=4
  Demux : Demux  Outputs=2
  Gain1 : Gain  Gain=1/ks
  Mux3 : Mux  Inputs=2
  PI_d1 : powerlib_extras/Discrete  Control Blocks/Discrete PI Controller  Kp=Kp(1)  Ki=Kp(2)  Par_Limits=[1 -1]*0.15  Init=0  Ts=Ts
  PI_d2 : powerlib_extras/Discrete  Control Blocks/Discrete PI Controller  Kp=Kd(1)  Ki=Kd(2)  Par_Limits=[1 -1]*0.25  Init=0  Ts=Ts
  Scope : Scope  NumInputPorts=2
  Subsystem1 : Subsystem
  Subtract : Sum  Inputs=+-
  Subtract1 : Sum
  Subtract2 : Sum  Inputs=+-
  Vdqref : Subsystem
  abc_dq : Subsystem
  abc_dq1 : Subsystem
  measure : Subsystem
  Vdqpu : Outport  VectorParamsAs1DForOutWhenUnconnected=off
  wires:
  Subtract2/1 -> measure/1(A=X-V)
  Subsystem1/1(Idqref) -> measure/2(Idqref), Subtract/1  "idqref"
  abc_dq/1(dq) -> Subtract2/2, Vdqref/1(Vdq2), Subsystem1/1(Vdq2)  "Vdq"
  abc_dq1/1(dq) -> Vdqref/2(Idqref), Subtract/2  "idq"
  Subtract/1 -> Scope/2, Demux/1
  Demux/1 -> PI_d2/1
  Demux/2 -> PI_d1/1
  Vdqref/1(Vdqrefss) -> Subtract1/1
  PI_d2/1 -> Mux3/1
  PI_d1/1 -> Mux3/2
  Mux3/1 -> Scope/1, Subtract1/2
  Subtract1/1 -> Subtract2/1, Gain1/1
  Vabcpu/1 -> abc_dq/1(abc)  "vabc"
  theda/1 -> abc_dq/2(theta), abc_dq1/2(theta)
  PQrefpu/1 -> Subsystem1/2(PQref)
  iabcpu/1 -> abc_dq1/1(abc)  "iabc"
  Gain1/1 -> Vdqpu/1  "Vdqpu"

== system RT_AI/SM_AI/Rec_VQcontrol2/pqctrl/dq->abc ==
  note: Va= Vd*sinwt + Vq*cos(wt) + Vo
  note: Vb= Vd*sin(wt-2pi/3) + Vq*cos(wt-2pi/3) + Vo
  note: Vc= Vd*sin(wt+2pi/3) + Vq*cos(wt+2pi/3) + Vo
  dq : Inport
  theda : Inport  Port=2
  Fcn : Fcn  Expr=(u(1)*sin(u(3))+u(2)*cos(u(3)))
  Fcn1 : Fcn  Expr=(u(1)*sin(u(3)-2*pi/3)+u(2)*cos(u(3)-2*pi/3))
  Fcn2 : Fcn  Expr=(u(1)*sin(u(3)+2*pi/3)+u(2)*cos(u(3)+2*pi/3))
  Mux1 : Mux  Inputs=2
  Mux3 : Mux  Inputs=3
  abc : Outport  VectorParamsAs1DForOutWhenUnconnected=off
  wires:
  Fcn2/1 -> Mux3/3
  Fcn1/1 -> Mux3/2
  Fcn/1 -> Mux3/1
  Mux1/1 -> Fcn/1, Fcn2/1, Fcn1/1
  dq/1 -> Mux1/1
  theda/1 -> Mux1/2
  Mux3/1 -> abc/1  "abc"

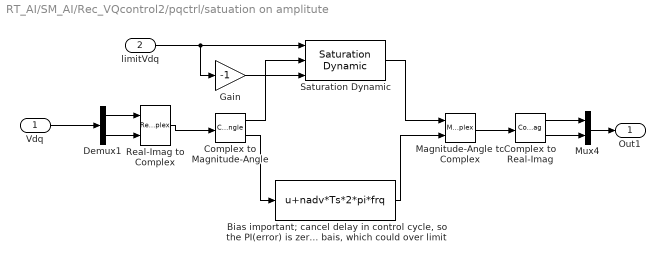
== system RT_AI/SM_AI/Rec_VQcontrol2/pqctrl/satuation on amplitute  ==
  Vdq : Inport
  limitVdq : Inport  Port=2
  "Bias important; cancel delay in control cycle, so the PI(error) is zero, other wise PI(errer) is bais, which could over limit" : Bias  Bias=nadv*Ts*2*pi*frq  SaturateOnIntegerOverflow=off
  Complex to Magnitude-Angle : ComplexToMagnitudeAngle
  Complex to Real-Imag : ComplexToRealImag
  Demux1 : Demux  Outputs=2
  Gain : Gain  Gain=-1
  Magnitude-Angle to Complex : MagnitudeAngleToComplex
  Mux4 : Mux  Inputs=2
  Real-Imag to Complex : RealImagToComplex
  Saturation Dynamic : simulink/Discontinuities/Saturation Dynamic  OutMin=[]  OutMax=[]  OutDataTypeStr=Inherit: Same as second input  OutDataType=fixdt(1, 16)  OutScaling=2^-10  DoSatur=off
  Out1 : Outport  VectorParamsAs1DForOutWhenUnconnected=off
  wires:
  "Bias important; cancel delay in control cycle, so the PI(error) is zero, other wise PI(errer) is bais, which could over limit"/1 -> Magnitude-Angle to Complex/2
  Gain/1 -> Saturation Dynamic/3
  limitVdq/1 -> Saturation Dynamic/1, Gain/1
  Complex to Magnitude-Angle/1 -> Saturation Dynamic/2
  Saturation Dynamic/1 -> Magnitude-Angle to Complex/1
  Demux1/1 -> Real-Imag to Complex/1
  Demux1/2 -> Real-Imag to Complex/2
  Real-Imag to Complex/1 -> Complex to Magnitude-Angle/1
  Complex to Magnitude-Angle/2 -> "Bias important; cancel delay in control cycle, so the PI(error) is zero, other wise PI(errer) is bais, which could over limit"/1
  Magnitude-Angle to Complex/1 -> Complex to Real-Imag/1
  Complex to Real-Imag/2 -> Mux4/2
  Complex to Real-Imag/1 -> Mux4/1
  Mux4/1 -> Out1/1
  Vdq/1 -> Demux1/1

== system RT_AI/SM_AI/Rec_VQcontrol2/Vdc ctrl/Vdc_ctrler1/PI_d2 ==
  note: Discrete PID Controller
  note: Pierre Giroux, Gilbert Sybille
      | Power System Simulation Laboratory
      | IREQ, Hydro-Quebc
  Error : Inport  SampleTime=Ts
  Discrete-Time Integrator : DiscreteIntegrator  InitialCondition=Init  SampleTime=Ts  LimitOutput=on  UpperSaturationLimit=UpperLimit  LowerSaturationLimit=LowerLimit  ICPrevOutput=DiscIntNeverNeededParam  ICPrevScaledInput=DiscIntNeverNeededParam
  Kp4 : Gain  Gain=Kp  SaturateOnIntegerOverflow=on  SampleTime=Ts  OutDataTypeStr=Inherit: Same as input  ParamDataTypeStr=Inherit: Same as input
  Kp5 : Gain  Gain=Ki  SaturateOnIntegerOverflow=on  SampleTime=Ts  OutDataTypeStr=Inherit: Same as input  ParamDataTypeStr=Inherit: Same as input
  Saturation2 : Saturate  UpperLimit=UpperLimit  LowerLimit=LowerLimit  SampleTime=Ts
  Sum6 : Sum  InputSameDT=on  SaturateOnIntegerOverflow=on  SampleTime=Ts  OutDataTypeStr=Inherit: Same as first input
  Zero-Order Hold : ZeroOrderHold  SampleTime=Ts
  Out : Outport  SampleTime=Ts  InitialOutput=0  VectorParamsAs1DForOutWhenUnconnected=off
  wires:
  Zero-Order Hold/1 -> Sum6/1  "prop"
  Saturation2/1 -> Out/1
  Discrete-Time Integrator/1 -> Sum6/2  "int"
  Kp4/1 -> Zero-Order Hold/1
  Kp5/1 -> Discrete-Time Integrator/1
  Sum6/1 -> Saturation2/1
  Error/1 -> Kp5/1, Kp4/1

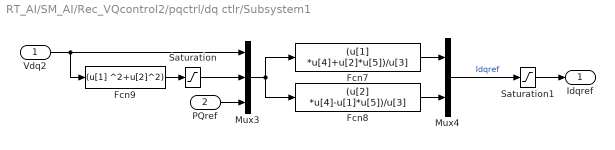
== system RT_AI/SM_AI/Rec_VQcontrol2/pqctrl/dq ctlr/Subsystem1 ==
  Vdq2 : Inport
  PQref : Inport  Port=2
  Fcn7 : Fcn  Expr=(u[1] *u[4]+u[2]*u[5])/u[3]
  Fcn8 : Fcn  Expr=(u[2] *u[4]-u[1]*u[5])/u[3]
  Fcn9 : Fcn  Expr=(u[1] ^2+u[2]^2)
  Mux3 : Mux  Inputs=[2 1 2]
  Mux4 : Mux  Inputs=2
  Saturation : Saturate  UpperLimit=inf  LowerLimit=0.01
  Saturation1 : Saturate  UpperLimit=1.5  LowerLimit=-1.5
  Idqref : Outport  VectorParamsAs1DForOutWhenUnconnected=off
  wires:
  Saturation1/1 -> Idqref/1
  Vdq2/1 -> Fcn9/1, Mux3/1
  Mux3/1 -> Fcn8/1, Fcn7/1
  Fcn9/1 -> Saturation/1
  Fcn7/1 -> Mux4/1
  Fcn8/1 -> Mux4/2
  Mux4/1 -> Saturation1/1  "Idqref"
  PQref/1 -> Mux3/3
  Saturation/1 -> Mux3/2

== system RT_AI/SM_AI/Rec_VQcontrol2/pqctrl/dq ctlr/Vdqref ==
  Vdq2 : Inport
  Idqref : Inport  Port=2
  Display : Display
      settings: Decimation=50
  Fcn7 : Fcn  Expr=(u[2] +u[4]*u[5]+u[3]*u[6])
  Fcn8 : Fcn  Expr=(u[1] +u[3]*u[5]-u[4]*u[6])
  Lxpu : Constant  Value=Lxpu
  Mux3 : Mux
  Mux4 : Mux  Inputs=2
  Rxpu : Constant  Value=Rxpu
  Vdqrefss : Outport  VectorParamsAs1DForOutWhenUnconnected=off
  wires:
  Lxpu/1 -> Mux3/4
  Rxpu/1 -> Mux3/3
  Mux3/1 -> Display/1, Fcn8/1, Fcn7/1
  Fcn8/1 -> Mux4/1  "Vdref"
  Fcn7/1 -> Mux4/2  "Vqref"
  Vdq2/1 -> Mux3/1
  Idqref/1 -> Mux3/2
  Mux4/1 -> Vdqrefss/1

== system RT_AI/SM_AI/Rec_VQcontrol2/pqctrl/dq ctlr/abc_dq ==
  abc : Inport
  theta : Inport  Port=2
  Mux2 : Mux  Inputs=2
  Selector3 : Selector  InputPortWidth=3  IndexOptions=Index vector (dialog)  Indices=[1 2]  OutputSizes=1
  Trigonometric Function2 : Trigonometry
  Trigonometric Function3 : Trigonometry  Operator=cos
  abc/dq1 : powerlib_extras/Measurements/abc_to_dq0 Transformation
  dq : Outport  VectorParamsAs1DForOutWhenUnconnected=off
  wires:
  abc/1 -> abc/dq1/1
  Selector3/1 -> dq/1
  abc/dq1/1 -> Selector3/1
  Mux2/1 -> abc/dq1/2
  theta/1 -> Trigonometric Function3/1, Trigonometric Function2/1
  Trigonometric Function2/1 -> Mux2/1
  Trigonometric Function3/1 -> Mux2/2

== system RT_AI/SM_AI/Rec_VQcontrol2/pqctrl/dq ctlr/abc_dq1 ==
  abc : Inport
  theta : Inport  Port=2
  Mux2 : Mux  Inputs=2
  Selector3 : Selector  InputPortWidth=3  IndexOptions=Index vector (dialog)  Indices=[1 2]  OutputSizes=1
  Trigonometric Function2 : Trigonometry
  Trigonometric Function3 : Trigonometry  Operator=cos
  abc/dq1 : powerlib_extras/Measurements/abc_to_dq0 Transformation
  dq : Outport  VectorParamsAs1DForOutWhenUnconnected=off
  wires:
  Trigonometric Function3/1 -> Mux2/2
  Trigonometric Function2/1 -> Mux2/1
  theta/1 -> Trigonometric Function2/1, Trigonometric Function3/1
  Mux2/1 -> abc/dq1/2
  abc/dq1/1 -> Selector3/1
  Selector3/1 -> dq/1
  abc/1 -> abc/dq1/1

== system RT_AI/SM_AI/Rec_VQcontrol2/pqctrl/dq ctlr/measure ==
  note: this is to validate Rxpu and Lxpu which make PI(error) almost zero,
      | i.e. the delay is properly set
      |
      | or to calculate Rxpu and Lxpu which make PI(error) zero
      | when input are in steady state
      |
      | when change the P,Q ref,
      | the results should be same if delay is properly cancelled
  A=X-V : Inport
  Idqref : Inport  Port=2
  Display1 : Display
      settings: Decimation=200
  Fcn7 : Fcn  Expr=(u[2] *u[3]-u[1]*u[4])/(u[3]^2+u[4]^2)
  Fcn8 : Fcn  Expr=(u[1] *u[3]+u[2]*u[4])/(u[3]^2+u[4]^2)
  Mux3 : Mux  Inputs=2
  Mux4 : Mux  Inputs=2
  wires:
  Mux3/1 -> Fcn8/1, Fcn7/1
  Fcn8/1 -> Mux4/1  "Rxpu"
  Fcn7/1 -> Mux4/2  "Lxpu"
  A=X-V/1 -> Mux3/1
  Idqref/1 -> Mux3/2
  Mux4/1 -> Display1/1

== matlab function RT_AI/SM_AI/MATLAB Function ==
  data: u input; dz output
function dz = phnode_forward(u)
    % =========================================================
    % 0. 声明持久化变量 (仅在 t=0 时加载和计算一次)
    % =========================================================
    persistent W00 b00 W01 b01 W10 b10 W11 b11 W20 b20 W21 b21 W3 b3 p
    
    if isempty(W00)

        w = coder.load('2level_pHNODE_weights.mat');
        
        W00 = double(w.R_module_net_0_0_weight); b00 = double(w.R_module_net_0_0_bias(:));
        W01 = double(w.R_module_net_0_1_weight(:)); b01 = double(w.R_module_net_0_1_bias(:));
        
        W10 = double(w.R_module_net_1_0_weight); b10 = double(w.R_module_net_1_0_bias(:));
        W11 = double(w.R_module_net_1_1_weight(:)); b11 = double(w.R_module_net_1_1_bias(:));
        
        W20 = double(w.R_module_net_2_0_weight); b20 = double(w.R_module_net_2_0_bias(:));
        W21 = double(w.R_module_net_2_1_weight(:)); b21 = double(w.R_module_net_2_1_bias(:));
        
        W3  = double(w.R_module_net_3_weight);   b3  = double(w.R_module_net_3_bias(:));

        p_raw = double(w.Pinv_module_p_raw(:));
        base_scale = [1/3.3e-3; 1/3.3e-3; 1/0.015; 1/0.015; 1/0.015];
        p = log(1.0 + exp(p_raw)) .* base_scale;
    end
    
    % =========================================================
    % 1. 拆解输入向量
    % =========================================================
    z     = double(u(1:5));
    u_ext = double(u(6:10));
    u_sw  = double(u(11:16));
    
    % =========================================================
    % 2. 构造耗散矩阵 R
    % =========================================================
    h = [z; u_sw];
    
    % --- Block 0 ---
    h = W00 * h + b00;
    mu = mean(h); var_h = mean((h - mu).^2);
    h = (h - mu) ./ sqrt(var_h + 1e-5);
    h = W01 .* h + b01;
    h = h ./ (1 + exp(-h)); % SiLU
    
    % --- Block 1 ---    
    h = W10 * h + b10;
    mu = mean(h); var_h = mean((h - mu).^2);
    h = (h - mu) ./ sqrt(var_h + 1e-5);
    h = W11 .* h + b11;
    h = h ./ (1 + exp(-h));
    
    % --- Block 2 ---
    h = W20 * h + b20;
    mu = mean(h); var_h = mean((h - mu).^2);
    h = (h - mu) ./ sqrt(var_h + 1e-5);
    h = W21 .* h + b21;
    h = h ./ (1 + exp(-h));
    
    % --- Output Linear ---
    r_out = W3 * h + b3;   
    r_full = log(1 + exp(r_out)); 
    
    % =========================================================
    % 3. 计算最终输出 dz 稀疏运算
    % =========================================================
    Jz = zeros(5, 1, 'double');
    Jz(1) =  u_sw(1)*z(3) + u_sw(3)*z(4) + u_sw(5)*z(5);
    Jz(2) = -u_sw(2)*z(3) - u_sw(4)*z(4) - u_sw(6)*z(5);
    Jz(3) = -u_sw(1)*z(1) + u_sw(2)*z(2);
    Jz(4) = -u_sw(3)*z(1) + u_sw(4)*z(2);
    Jz(5) = -u_sw(5)*z(1) + u_sw(6)*z(2);
 
    rhs = Jz - r_full .* z + u_ext;
 
    dz = p .* rhs;
end

== matlab function RT_AI/SM_AI/MATLAB Function1 ==
  settings: updateMethod=DISCRETE
  data: u input; dz output
function dz = phnode_forward(u)
    % =========================================================
    % 0. 声明持久化变量 (仅在 t=0 时加载和计算一次)
    % =========================================================
    persistent W00 b00 W01 b01 W10 b10 W11 b11 W20 b20 W21 b21 W3 b3 p
    
    if isempty(W00)

        w = coder.load('2level_pHNODE_weights.mat');
        
        W00 = double(w.R_module_net_0_0_weight); b00 = double(w.R_module_net_0_0_bias(:));
        W01 = double(w.R_module_net_0_1_weight(:)); b01 = double(w.R_module_net_0_1_bias(:));
        
        W10 = double(w.R_module_net_1_0_weight); b10 = double(w.R_module_net_1_0_bias(:));
        W11 = double(w.R_module_net_1_1_weight(:)); b11 = double(w.R_module_net_1_1_bias(:));
        
        W20 = double(w.R_module_net_2_0_weight); b20 = double(w.R_module_net_2_0_bias(:));
        W21 = double(w.R_module_net_2_1_weight(:)); b21 = double(w.R_module_net_2_1_bias(:));
        
        W3  = double(w.R_module_net_3_weight);   b3  = double(w.R_module_net_3_bias(:));

        p_raw = double(w.Pinv_module_p_raw(:));
        base_scale = [1/3.3e-3; 1/3.3e-3; 1/0.015; 1/0.015; 1/0.015];
        p = log(1.0 + exp(p_raw)) .* base_scale;
    end
    
    % =========================================================
    % 1. 拆解输入向量
    % =========================================================
    z     = double(u(1:5));
    u_ext = double(u(6:10));
    u_sw  = double(u(11:16));
    
    % =========================================================
    % 2. 构造耗散矩阵 R
    % =========================================================
    h = [z; u_sw];
    
    % --- Block 0 ---
    h = W00 * h + b00;
    mu = mean(h); var_h = mean((h - mu).^2);
    h = (h - mu) ./ sqrt(var_h + 1e-5);
    h = W01 .* h + b01;
    h = h ./ (1 + exp(-h)); % SiLU
    
    % --- Block 1 ---    
    h = W10 * h + b10;
    mu = mean(h); var_h = mean((h - mu).^2);
    h = (h - mu) ./ sqrt(var_h + 1e-5);
    h = W11 .* h + b11;
    h = h ./ (1 + exp(-h));
    
    % --- Block 2 ---
    h = W20 * h + b20;
    mu = mean(h); var_h = mean((h - mu).^2);
    h = (h - mu) ./ sqrt(var_h + 1e-5);
    h = W21 .* h + b21;
    h = h ./ (1 + exp(-h));
    
    % --- Output Linear ---
    r_out = W3 * h + b3;   
    r_full = log(1 + exp(r_out)); 
    
    % =========================================================
    % 3. 计算最终输出 dz 稀疏运算
    % =========================================================
    Jz = zeros(5, 1, 'double');
    Jz(1) =  u_sw(1)*z(3) + u_sw(3)*z(4) + u_sw(5)*z(5);
    Jz(2) = -u_sw(2)*z(3) - u_sw(4)*z(4) - u_sw(6)*z(5);
    Jz(3) = -u_sw(1)*z(1) + u_sw(2)*z(2);
    Jz(4) = -u_sw(3)*z(1) + u_sw(4)*z(2);
    Jz(5) = -u_sw(5)*z(1) + u_sw(6)*z(2);
 
    rhs = Jz - r_full .* z + u_ext;
 
    dz = p .* rhs;
end
